simulink model "cdcon"  (R2023a)
settings: Solver=ode23t  StartTime=0.0  StopTime=0.005  RelTol=1e-3
values from neighbouring files (symbols this model uses):
  C = 0.00001    (= 1e-05)    [BUCK.m]    (also in DIF.m = [c1 -m2*l2*x(4)*sin(x(2)-x(1));l1*x(3)*sin(x(2)-x(1)) 0])
  L = 0.002    [BUCK.m]
  R = 10    [BUCK.m]
  U = 32    [BUCK.m]
settings Model: Creator=edgar  LastModifiedBy=erick
settings OptimizationCC: ReuseModelBlockBuffer=off

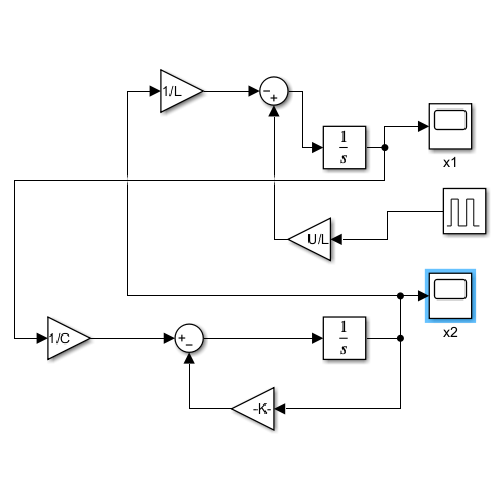
[thumbnail: Simulink's stored preview of the top-level diagram]
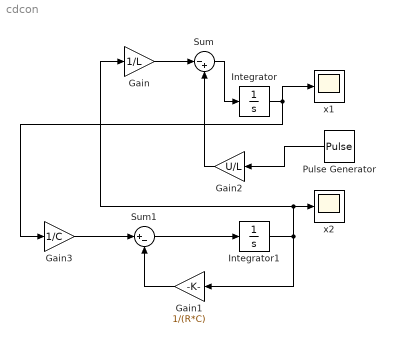
== system cdcon ==
  Gain : Gain  Gain=1/L
  Gain1 : Gain  Gain=1/(R*C)
  Gain2 : Gain  Gain=U/L
  Gain3 : Gain  Gain=1/C
  Integrator : Integrator
  Integrator1 : Integrator
  Pulse Generator : DiscretePulseGenerator  PulseType=Time based  Amplitude=0.955  Period=1e-5  PulseWidth=40
  Sum : Sum  Inputs=|-+
  Sum1 : Sum  Inputs=|+-
  x1 : Scope
  x2 : Scope
  wires:
  Sum/1 -> Integrator/1
  Gain/1 -> Sum/1
  Sum1/1 -> Integrator1/1
  Integrator1/1 -> x2/1, Gain/1, Gain1/1
  Gain2/1 -> Sum/2
  Gain1/1 -> Sum1/2
  Gain3/1 -> Sum1/1
  Integrator/1 -> x1/1, Gain3/1
  Pulse Generator/1 -> Gain2/1
